simulink model "Pi_LUPA"  (R2024b)
settings: Solver=VariableStepAuto  StartTime=0.0  StopTime=t_stop  RelTol=1e-3
values from neighbouring files (symbols this model uses):
  C = 1.97e3/2    (= 985)    [general_pi_init.m]
  L = 5.21e-5    (= 5.21e-05)    [general_pi_init.m]
  SIL = sqrt(L/C)    [general_pi_init.m]
  T = table(freqs.', peak_ts.', peak_abk.', peak_conv.',      'VariableNames', {'Frequency_Hz','Peak_WAMIT_N','Peak_ABK_N','Peak_Conv_N'})    [F_ex_appx.m]    (also in general_pi_init.m = 10)
undefined symbols (not defined in the file or in its folder): A, ckt, dspblkCoreblockFVToolHelper, gcbh, IRF_dt, wd
libraries: fl_lib x229, nesl_utility x133, simulink x4, ee_lib x1
(part 1 of 4)
settings Model: Creator=inyongkim  LastModifiedBy=inyongkim

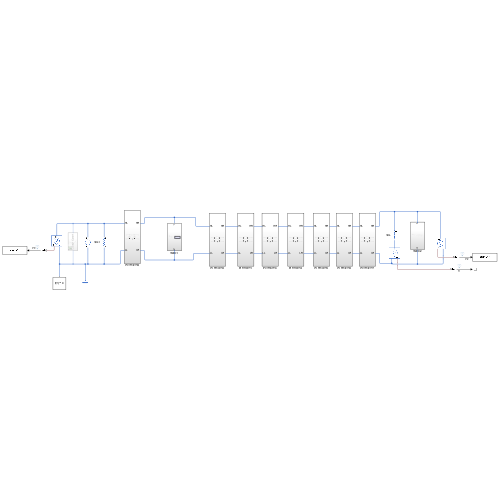
[thumbnail: Simulink's stored preview of the top-level diagram]
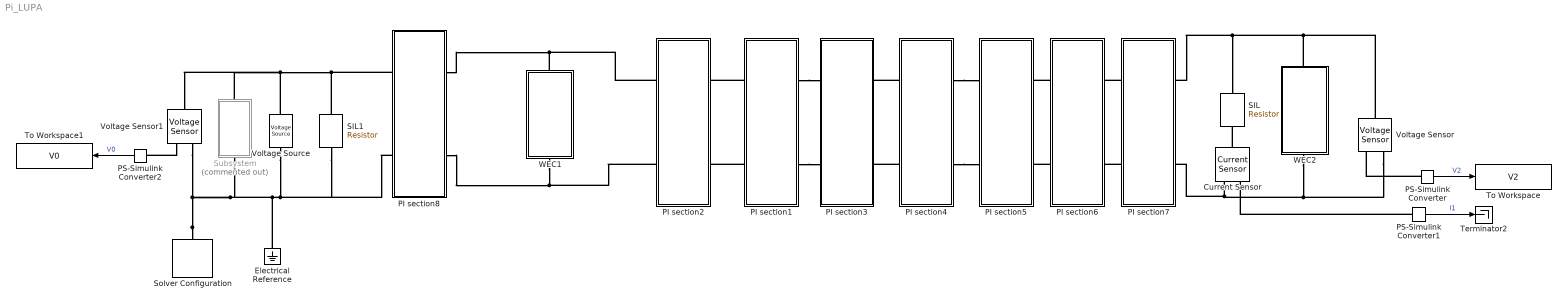
== system Pi_LUPA ==
  Current Sensor : fl_lib/Electrical/Electrical Sensors/Current Sensor
  Electrical Reference : fl_lib/Electrical/Electrical Elements/Electrical Reference
  PI section1 : Subsystem
  PI section2 : Subsystem
  PI section3 : Subsystem
  PI section4 : Subsystem
  PI section5 : Subsystem
  PI section6 : Subsystem
  PI section7 : Subsystem
  PI section8 : Subsystem
  PS-Simulink Converter : nesl_utility/PS-Simulink Converter  PhysicalDomain=network_engine_domain  SubClassName=ps_output  LeftPortType=input  RightPortType=output  PseudoPeriodic=off  Frequencies=[]  VectorFormat=inherit  Unit=inherit  AffineConversion=off
  PS-Simulink Converter1 : nesl_utility/PS-Simulink Converter  PhysicalDomain=network_engine_domain  SubClassName=ps_output  LeftPortType=input  RightPortType=output  PseudoPeriodic=off  Frequencies=[]  VectorFormat=inherit  Unit=inherit  AffineConversion=off
  PS-Simulink Converter2 : nesl_utility/PS-Simulink Converter  PhysicalDomain=network_engine_domain  SubClassName=ps_output  LeftPortType=input  RightPortType=output  PseudoPeriodic=off  Frequencies=[]  VectorFormat=inherit  Unit=inherit  AffineConversion=off
  SIL : fl_lib/Electrical/Electrical Elements/Resistor  R=SIL Ohm  i_specify=off  i_priority=None  i=0 A  i_nominal_specify=off  i_nominal_value=1  i_nominal_unit=A  v_specify=off  v_priority=None  v=0 V  v_nominal_specify=off  v_nominal_value=1  v_nominal_unit=V
  SIL1 : fl_lib/Electrical/Electrical Elements/Resistor  R=SIL*1e6 Ohm  i_specify=off  i_priority=None  i=0 A  i_nominal_specify=off  i_nominal_value=1  i_nominal_unit=A  v_specify=off  v_priority=None  v=0 V  v_nominal_specify=off  v_nominal_value=1  v_nominal_unit=V
  Solver Configuration : nesl_utility/Solver Configuration  PhysicalDomain=network_engine_domain  SubClassName=solver  LeftPortType=input  RightPortType=generic  Tones=[]  Harmonics=[]  SimulateNoise=off  Profile=off  UseLocalSampling=off  EnableSwitchedLinearOptims=on  FrequencyDomain=off  UseCCode=off  RelTol=0.001  AbsTol=0.001  MinStep=1e-09  ToWorkspace=off  RevertToSquareIcSolve=off  NumHomotopyIterations=100  PhasorMode=off  PhasorModeNumHarmonics=1  ConsistencySolver=NEWTON_XTOL_AFTER_FTOL  IndexReductionMethod=None  DoDC=off  ResidualTolerance=1e-09  ConsistencyTolSource=GLOBAL  ConsistencyAbsTol=0.001  ConsistencyRelTol=0.001  ConsistencyTolFactor=0.001  UseLocalSolver=off  LocalSolverChoice=NE_BACKWARD_EULER_ADVANCER  ResolveIndetEquations=on  FunctionEvalNumThread=1  LocalSolverSampleTime=0.001  DoFixedCost=off  MaxNonlinIter=3  MaxModeIter=2  ComputeImpulses=off  ImpulseIterations=2  LinearAlgebra=auto  LinearAlgebraNumThread=0  EquationFormulation=NE_TIME_EF  DelaysMemoryBudget=1024  AutomaticFiltering=on  FilteringTimeConstant=0.001  PartitionStorageMethod=AS_NEEDED  PartitionMemoryBudget=1024  PartitionMethod=ROBUST  MultibodyUseLocalSolver=off  MultibodyLocalSolverChoice=ODE1  MultibodyLocalSolverSampleTime=0.001
  Subsystem : Subsystem  Commented=on
  Terminator2 : Terminator
  To Workspace : ToWorkspace  VariableName=V2  SaveFormat=Timeseries  SampleTime=-1
  To Workspace1 : ToWorkspace  VariableName=V0  SaveFormat=Timeseries  SampleTime=-1
  Voltage Sensor : fl_lib/Electrical/Electrical Sensors/Voltage Sensor
  Voltage Sensor1 : fl_lib/Electrical/Electrical Sensors/Voltage Sensor
  Voltage Source : ee_lib/Sources/Voltage Source  dc_voltage=0 V  ac_voltage=A*2*pi/T V  ac_shift=0 rad  ac_frequency=1/T Hz  noise_mode=ee.enum.sources.noise.Disabled  PSD=0 V^2/Hz  sample_time=1e-3 s  repeatability=ee.enum.sources.repeatability.NotRepeatable  user_seed=0  auto_seed=3010019299  i_specify=off  i_priority=None  i=0 A  i_nominal_specify=off  i_nominal_value=1  i_nominal_unit=A  v_specify=off  v_priority=None  v=0 V  v_nominal_specify=off  v_nominal_value=1  v_nominal_unit=V
  WEC1 : Subsystem
      settings: PortSchema="{\"entries\":[{\"content\":{\"sides\":[{\"content\":{},\"type\":\"ConnectorPlacement.EquallySpacedRectSide\",\"uuid\":\"610af32e-2de7-4c50-99be-cfe133541e3f\"},{\"content\":{\"side\":\"RIGHT\"},\"type\":\"ConnectorPlacement.EquallySpacedRectSide\",\"uuid\":\"0415963f-e440-414e-b6ca-8ae2fc36710b\"},{\"content\":{\"connectorIds\":[\"LConn1\"],\"side\":\"TOP\"},\"type\":\"ConnectorPlacement.EquallySpacedRectSide\",\"uuid\":\"323fcf80-8c19-453d-8de3-ca4665704952\"},{\"content\":{\"connectorIds\":[\"RConn1\"],\"side\":\"BOTTOM\"},\"type\":\"ConnectorPlacement.EquallySpacedRectSide\",\"uuid\":\"a977eb3e-c443-4e6c-8731-998188d6bcfb\"}]},\"type\":\"ConnectorPlacement.EquallySpacedConnector\",\"uuid\":\"11f40d62-75d3-4550-8fc4-6982ab3d84ea\"}],\"packageUris\":[\"http://schema.mathworks.com/mf0/Connector/R2020b\"],\"version\":\"1.0\"}"
  WEC2 : Subsystem
      settings: PortSchema="{\"entries\":[{\"content\":{\"sides\":[{\"content\":{},\"type\":\"ConnectorPlacement.EquallySpacedRectSide\",\"uuid\":\"610af32e-2de7-4c50-99be-cfe133541e3f\"},{\"content\":{\"side\":\"RIGHT\"},\"type\":\"ConnectorPlacement.EquallySpacedRectSide\",\"uuid\":\"0415963f-e440-414e-b6ca-8ae2fc36710b\"},{\"content\":{\"connectorIds\":[\"LConn1\"],\"side\":\"TOP\"},\"type\":\"ConnectorPlacement.EquallySpacedRectSide\",\"uuid\":\"323fcf80-8c19-453d-8de3-ca4665704952\"},{\"content\":{\"connectorIds\":[\"RConn1\"],\"side\":\"BOTTOM\"},\"type\":\"ConnectorPlacement.EquallySpacedRectSide\",\"uuid\":\"a977eb3e-c443-4e6c-8731-998188d6bcfb\"}]},\"type\":\"ConnectorPlacement.EquallySpacedConnector\",\"uuid\":\"11f40d62-75d3-4550-8fc4-6982ab3d84ea\"}],\"packageUris\":[\"http://schema.mathworks.com/mf0/Connector/R2020b\"],\"version\":\"1.0\"}"
  wires:
  PS-Simulink Converter/1 -> To Workspace/1  "V2"
  PS-Simulink Converter1/1 -> Terminator2/1  "I1"
  PS-Simulink Converter2/1 -> To Workspace1/1  "V0"
  connections:
  Solver Configuration/RConn1 -- Subsystem/RConn1 -- Voltage Source/RConn1 -- SIL1/RConn1 -- PI section8/LConn2 -- Electrical Reference/LConn1 -- Voltage Sensor1/RConn2
  Voltage Source/LConn1 -- Subsystem/LConn1 -- Voltage Sensor1/LConn1 -- SIL1/LConn1 -- PI section8/LConn1
  Voltage Sensor/LConn1 -- WEC2/LConn1 -- SIL/LConn1 -- PI section7/RConn1
  PS-Simulink Converter/LConn1 -- Voltage Sensor/RConn1
  Current Sensor/LConn1 -- SIL/RConn1
  PS-Simulink Converter1/LConn1 -- Current Sensor/RConn1
  Voltage Sensor1/RConn1 -- PS-Simulink Converter2/LConn1
  WEC1/LConn1 -- PI section2/LConn1 -- PI section8/RConn1
  WEC1/RConn1 -- PI section2/LConn2 -- PI section8/RConn2
  Voltage Sensor/RConn2 -- WEC2/RConn1 -- PI section7/RConn2 -- Current Sensor/RConn2
  PI section1/RConn1 -- PI section3/LConn1
  PI section1/RConn2 -- PI section3/LConn2
  PI section4/LConn1 -- PI section3/RConn1
  PI section4/LConn2 -- PI section3/RConn2
  PI section4/RConn2 -- PI section5/LConn2
  PI section4/RConn1 -- PI section5/LConn1
  PI section6/LConn1 -- PI section5/RConn1
  PI section6/LConn2 -- PI section5/RConn2
  PI section1/LConn1 -- PI section2/RConn1
  PI section1/LConn2 -- PI section2/RConn2
  PI section7/LConn1 -- PI section6/RConn1
  PI section7/LConn2 -- PI section6/RConn2

== system Pi_LUPA/PI section1 ==
  Electrical Reference : fl_lib/Electrical/Electrical Elements/Electrical Reference
  General C : Subsystem
      settings: PortSchema="{\"entries\":[{\"content\":{\"sides\":[{\"content\":{},\"type\":\"ConnectorPlacement.EquallySpacedRectSide\",\"uuid\":\"54c7c027-76dd-4589-a14d-62021aaba10d\"},{\"content\":{\"side\":\"RIGHT\"},\"type\":\"ConnectorPlacement.EquallySpacedRectSide\",\"uuid\":\"5fae45fc-fbd0-44d0-9d3d-94b3e56c48e3\"},{\"content\":{\"connectorIds\":[\"LConn1\"],\"side\":\"TOP\"},\"type\":\"ConnectorPlacement.EquallySpacedRectSide\",\"uuid\":\"b6847d7e-9825-46ad-84aa-5df9156d119d\"},{\"content\":{\"connectorIds\":[\"RConn1\"],\"side\":\"BOTTOM\"},\"type\":\"ConnectorPlacement.EquallySpacedRectSide\",\"uuid\":\"1394d42d-8985-4309-a3e0-31ed6b8c9496\"}]},\"type\":\"ConnectorPlacement.EquallySpacedConnector\",\"uuid\":\"6a4af355-2598-47af-9220-e6e09375ad72\"}],\"packageUris\":[\"http://schema.mathworks.com/mf0/Connector/R2020b\"],\"version\":\"1.0\"}"
  General C1 : Subsystem
      settings: PortSchema="{\"entries\":[{\"content\":{\"sides\":[{\"content\":{},\"type\":\"ConnectorPlacement.EquallySpacedRectSide\",\"uuid\":\"54c7c027-76dd-4589-a14d-62021aaba10d\"},{\"content\":{\"side\":\"RIGHT\"},\"type\":\"ConnectorPlacement.EquallySpacedRectSide\",\"uuid\":\"5fae45fc-fbd0-44d0-9d3d-94b3e56c48e3\"},{\"content\":{\"connectorIds\":[\"LConn1\"],\"side\":\"TOP\"},\"type\":\"ConnectorPlacement.EquallySpacedRectSide\",\"uuid\":\"b6847d7e-9825-46ad-84aa-5df9156d119d\"},{\"content\":{\"connectorIds\":[\"RConn1\"],\"side\":\"BOTTOM\"},\"type\":\"ConnectorPlacement.EquallySpacedRectSide\",\"uuid\":\"1394d42d-8985-4309-a3e0-31ed6b8c9496\"}]},\"type\":\"ConnectorPlacement.EquallySpacedConnector\",\"uuid\":\"6a4af355-2598-47af-9220-e6e09375ad72\"}],\"packageUris\":[\"http://schema.mathworks.com/mf0/Connector/R2020b\"],\"version\":\"1.0\"}"
  General L : Subsystem
      settings: PortSchema="{\"entries\":[{\"content\":{\"sides\":[{\"content\":{},\"type\":\"ConnectorPlacement.EquallySpacedRectSide\",\"uuid\":\"54c7c027-76dd-4589-a14d-62021aaba10d\"},{\"content\":{\"side\":\"RIGHT\"},\"type\":\"ConnectorPlacement.EquallySpacedRectSide\",\"uuid\":\"5fae45fc-fbd0-44d0-9d3d-94b3e56c48e3\"},{\"content\":{\"connectorIds\":[\"LConn1\"],\"side\":\"TOP\"},\"type\":\"ConnectorPlacement.EquallySpacedRectSide\",\"uuid\":\"b6847d7e-9825-46ad-84aa-5df9156d119d\"},{\"content\":{\"connectorIds\":[\"RConn1\"],\"side\":\"BOTTOM\"},\"type\":\"ConnectorPlacement.EquallySpacedRectSide\",\"uuid\":\"7b301271-0a77-4acb-8843-591cb23b0585\"}]},\"type\":\"ConnectorPlacement.EquallySpacedConnector\",\"uuid\":\"6a4af355-2598-47af-9220-e6e09375ad72\"}],\"packageUris\":[\"http://schema.mathworks.com/mf0/Connector/R2020b\"],\"version\":\"1.0\"}"
  HL : PMIOPort  Side=Left
  HR : PMIOPort  Port=2  Side=Right
  LL : PMIOPort  Port=3  Side=Left
  LR : PMIOPort  Port=4  Side=Right
  connections:
  HL/RConn1 -- General L/LConn1 -- General C/LConn1
  General C/RConn1 -- LL/RConn1 -- Electrical Reference/LConn1 -- General C1/RConn1 -- LR/RConn1
  HR/RConn1 -- General C1/LConn1 -- General L/RConn1

== system Pi_LUPA/PI section2 ==
  Electrical Reference : fl_lib/Electrical/Electrical Elements/Electrical Reference
  General C : Subsystem
      settings: PortSchema="{\"entries\":[{\"content\":{\"sides\":[{\"content\":{},\"type\":\"ConnectorPlacement.EquallySpacedRectSide\",\"uuid\":\"54c7c027-76dd-4589-a14d-62021aaba10d\"},{\"content\":{\"side\":\"RIGHT\"},\"type\":\"ConnectorPlacement.EquallySpacedRectSide\",\"uuid\":\"5fae45fc-fbd0-44d0-9d3d-94b3e56c48e3\"},{\"content\":{\"connectorIds\":[\"LConn1\"],\"side\":\"TOP\"},\"type\":\"ConnectorPlacement.EquallySpacedRectSide\",\"uuid\":\"b6847d7e-9825-46ad-84aa-5df9156d119d\"},{\"content\":{\"connectorIds\":[\"RConn1\"],\"side\":\"BOTTOM\"},\"type\":\"ConnectorPlacement.EquallySpacedRectSide\",\"uuid\":\"1394d42d-8985-4309-a3e0-31ed6b8c9496\"}]},\"type\":\"ConnectorPlacement.EquallySpacedConnector\",\"uuid\":\"6a4af355-2598-47af-9220-e6e09375ad72\"}],\"packageUris\":[\"http://schema.mathworks.com/mf0/Connector/R2020b\"],\"version\":\"1.0\"}"
  General C1 : Subsystem
      settings: PortSchema="{\"entries\":[{\"content\":{\"sides\":[{\"content\":{},\"type\":\"ConnectorPlacement.EquallySpacedRectSide\",\"uuid\":\"54c7c027-76dd-4589-a14d-62021aaba10d\"},{\"content\":{\"side\":\"RIGHT\"},\"type\":\"ConnectorPlacement.EquallySpacedRectSide\",\"uuid\":\"5fae45fc-fbd0-44d0-9d3d-94b3e56c48e3\"},{\"content\":{\"connectorIds\":[\"LConn1\"],\"side\":\"TOP\"},\"type\":\"ConnectorPlacement.EquallySpacedRectSide\",\"uuid\":\"b6847d7e-9825-46ad-84aa-5df9156d119d\"},{\"content\":{\"connectorIds\":[\"RConn1\"],\"side\":\"BOTTOM\"},\"type\":\"ConnectorPlacement.EquallySpacedRectSide\",\"uuid\":\"1394d42d-8985-4309-a3e0-31ed6b8c9496\"}]},\"type\":\"ConnectorPlacement.EquallySpacedConnector\",\"uuid\":\"6a4af355-2598-47af-9220-e6e09375ad72\"}],\"packageUris\":[\"http://schema.mathworks.com/mf0/Connector/R2020b\"],\"version\":\"1.0\"}"
  General L : Subsystem
      settings: PortSchema="{\"entries\":[{\"content\":{\"sides\":[{\"content\":{},\"type\":\"ConnectorPlacement.EquallySpacedRectSide\",\"uuid\":\"54c7c027-76dd-4589-a14d-62021aaba10d\"},{\"content\":{\"side\":\"RIGHT\"},\"type\":\"ConnectorPlacement.EquallySpacedRectSide\",\"uuid\":\"5fae45fc-fbd0-44d0-9d3d-94b3e56c48e3\"},{\"content\":{\"connectorIds\":[\"LConn1\"],\"side\":\"TOP\"},\"type\":\"ConnectorPlacement.EquallySpacedRectSide\",\"uuid\":\"b6847d7e-9825-46ad-84aa-5df9156d119d\"},{\"content\":{\"connectorIds\":[\"RConn1\"],\"side\":\"BOTTOM\"},\"type\":\"ConnectorPlacement.EquallySpacedRectSide\",\"uuid\":\"7b301271-0a77-4acb-8843-591cb23b0585\"}]},\"type\":\"ConnectorPlacement.EquallySpacedConnector\",\"uuid\":\"6a4af355-2598-47af-9220-e6e09375ad72\"}],\"packageUris\":[\"http://schema.mathworks.com/mf0/Connector/R2020b\"],\"version\":\"1.0\"}"
  HL : PMIOPort  Side=Left
  HR : PMIOPort  Port=2  Side=Right
  LL : PMIOPort  Port=3  Side=Left
  LR : PMIOPort  Port=4  Side=Right
  connections:
  General L/RConn1 -- General C1/LConn1 -- HR/RConn1
  LR/RConn1 -- Electrical Reference/LConn1 -- LL/RConn1 -- General C/RConn1 -- General C1/RConn1
  General C/LConn1 -- General L/LConn1 -- HL/RConn1

== system Pi_LUPA/PI section3 ==
  Electrical Reference : fl_lib/Electrical/Electrical Elements/Electrical Reference
  General C : Subsystem
      settings: PortSchema="{\"entries\":[{\"content\":{\"sides\":[{\"content\":{},\"type\":\"ConnectorPlacement.EquallySpacedRectSide\",\"uuid\":\"54c7c027-76dd-4589-a14d-62021aaba10d\"},{\"content\":{\"side\":\"RIGHT\"},\"type\":\"ConnectorPlacement.EquallySpacedRectSide\",\"uuid\":\"5fae45fc-fbd0-44d0-9d3d-94b3e56c48e3\"},{\"content\":{\"connectorIds\":[\"LConn1\"],\"side\":\"TOP\"},\"type\":\"ConnectorPlacement.EquallySpacedRectSide\",\"uuid\":\"b6847d7e-9825-46ad-84aa-5df9156d119d\"},{\"content\":{\"connectorIds\":[\"RConn1\"],\"side\":\"BOTTOM\"},\"type\":\"ConnectorPlacement.EquallySpacedRectSide\",\"uuid\":\"1394d42d-8985-4309-a3e0-31ed6b8c9496\"}]},\"type\":\"ConnectorPlacement.EquallySpacedConnector\",\"uuid\":\"6a4af355-2598-47af-9220-e6e09375ad72\"}],\"packageUris\":[\"http://schema.mathworks.com/mf0/Connector/R2020b\"],\"version\":\"1.0\"}"
  General C1 : Subsystem
      settings: PortSchema="{\"entries\":[{\"content\":{\"sides\":[{\"content\":{},\"type\":\"ConnectorPlacement.EquallySpacedRectSide\",\"uuid\":\"54c7c027-76dd-4589-a14d-62021aaba10d\"},{\"content\":{\"side\":\"RIGHT\"},\"type\":\"ConnectorPlacement.EquallySpacedRectSide\",\"uuid\":\"5fae45fc-fbd0-44d0-9d3d-94b3e56c48e3\"},{\"content\":{\"connectorIds\":[\"LConn1\"],\"side\":\"TOP\"},\"type\":\"ConnectorPlacement.EquallySpacedRectSide\",\"uuid\":\"b6847d7e-9825-46ad-84aa-5df9156d119d\"},{\"content\":{\"connectorIds\":[\"RConn1\"],\"side\":\"BOTTOM\"},\"type\":\"ConnectorPlacement.EquallySpacedRectSide\",\"uuid\":\"1394d42d-8985-4309-a3e0-31ed6b8c9496\"}]},\"type\":\"ConnectorPlacement.EquallySpacedConnector\",\"uuid\":\"6a4af355-2598-47af-9220-e6e09375ad72\"}],\"packageUris\":[\"http://schema.mathworks.com/mf0/Connector/R2020b\"],\"version\":\"1.0\"}"
  General L : Subsystem
      settings: PortSchema="{\"entries\":[{\"content\":{\"sides\":[{\"content\":{},\"type\":\"ConnectorPlacement.EquallySpacedRectSide\",\"uuid\":\"54c7c027-76dd-4589-a14d-62021aaba10d\"},{\"content\":{\"side\":\"RIGHT\"},\"type\":\"ConnectorPlacement.EquallySpacedRectSide\",\"uuid\":\"5fae45fc-fbd0-44d0-9d3d-94b3e56c48e3\"},{\"content\":{\"connectorIds\":[\"LConn1\"],\"side\":\"TOP\"},\"type\":\"ConnectorPlacement.EquallySpacedRectSide\",\"uuid\":\"b6847d7e-9825-46ad-84aa-5df9156d119d\"},{\"content\":{\"connectorIds\":[\"RConn1\"],\"side\":\"BOTTOM\"},\"type\":\"ConnectorPlacement.EquallySpacedRectSide\",\"uuid\":\"7b301271-0a77-4acb-8843-591cb23b0585\"}]},\"type\":\"ConnectorPlacement.EquallySpacedConnector\",\"uuid\":\"6a4af355-2598-47af-9220-e6e09375ad72\"}],\"packageUris\":[\"http://schema.mathworks.com/mf0/Connector/R2020b\"],\"version\":\"1.0\"}"
  HL : PMIOPort  Side=Left
  HR : PMIOPort  Port=2  Side=Right
  LL : PMIOPort  Port=3  Side=Left
  LR : PMIOPort  Port=4  Side=Right
  connections:
  General L/RConn1 -- General C1/LConn1 -- HR/RConn1
  LR/RConn1 -- Electrical Reference/LConn1 -- LL/RConn1 -- General C/RConn1 -- General C1/RConn1
  General C/LConn1 -- General L/LConn1 -- HL/RConn1

== system Pi_LUPA/PI section4 ==
  Electrical Reference : fl_lib/Electrical/Electrical Elements/Electrical Reference
  General C : Subsystem
      settings: PortSchema="{\"entries\":[{\"content\":{\"sides\":[{\"content\":{},\"type\":\"ConnectorPlacement.EquallySpacedRectSide\",\"uuid\":\"54c7c027-76dd-4589-a14d-62021aaba10d\"},{\"content\":{\"side\":\"RIGHT\"},\"type\":\"ConnectorPlacement.EquallySpacedRectSide\",\"uuid\":\"5fae45fc-fbd0-44d0-9d3d-94b3e56c48e3\"},{\"content\":{\"connectorIds\":[\"LConn1\"],\"side\":\"TOP\"},\"type\":\"ConnectorPlacement.EquallySpacedRectSide\",\"uuid\":\"b6847d7e-9825-46ad-84aa-5df9156d119d\"},{\"content\":{\"connectorIds\":[\"RConn1\"],\"side\":\"BOTTOM\"},\"type\":\"ConnectorPlacement.EquallySpacedRectSide\",\"uuid\":\"1394d42d-8985-4309-a3e0-31ed6b8c9496\"}]},\"type\":\"ConnectorPlacement.EquallySpacedConnector\",\"uuid\":\"6a4af355-2598-47af-9220-e6e09375ad72\"}],\"packageUris\":[\"http://schema.mathworks.com/mf0/Connector/R2020b\"],\"version\":\"1.0\"}"
  General C1 : Subsystem
      settings: PortSchema="{\"entries\":[{\"content\":{\"sides\":[{\"content\":{},\"type\":\"ConnectorPlacement.EquallySpacedRectSide\",\"uuid\":\"54c7c027-76dd-4589-a14d-62021aaba10d\"},{\"content\":{\"side\":\"RIGHT\"},\"type\":\"ConnectorPlacement.EquallySpacedRectSide\",\"uuid\":\"5fae45fc-fbd0-44d0-9d3d-94b3e56c48e3\"},{\"content\":{\"connectorIds\":[\"LConn1\"],\"side\":\"TOP\"},\"type\":\"ConnectorPlacement.EquallySpacedRectSide\",\"uuid\":\"b6847d7e-9825-46ad-84aa-5df9156d119d\"},{\"content\":{\"connectorIds\":[\"RConn1\"],\"side\":\"BOTTOM\"},\"type\":\"ConnectorPlacement.EquallySpacedRectSide\",\"uuid\":\"1394d42d-8985-4309-a3e0-31ed6b8c9496\"}]},\"type\":\"ConnectorPlacement.EquallySpacedConnector\",\"uuid\":\"6a4af355-2598-47af-9220-e6e09375ad72\"}],\"packageUris\":[\"http://schema.mathworks.com/mf0/Connector/R2020b\"],\"version\":\"1.0\"}"
  General L : Subsystem
      settings: PortSchema="{\"entries\":[{\"content\":{\"sides\":[{\"content\":{},\"type\":\"ConnectorPlacement.EquallySpacedRectSide\",\"uuid\":\"54c7c027-76dd-4589-a14d-62021aaba10d\"},{\"content\":{\"side\":\"RIGHT\"},\"type\":\"ConnectorPlacement.EquallySpacedRectSide\",\"uuid\":\"5fae45fc-fbd0-44d0-9d3d-94b3e56c48e3\"},{\"content\":{\"connectorIds\":[\"LConn1\"],\"side\":\"TOP\"},\"type\":\"ConnectorPlacement.EquallySpacedRectSide\",\"uuid\":\"b6847d7e-9825-46ad-84aa-5df9156d119d\"},{\"content\":{\"connectorIds\":[\"RConn1\"],\"side\":\"BOTTOM\"},\"type\":\"ConnectorPlacement.EquallySpacedRectSide\",\"uuid\":\"7b301271-0a77-4acb-8843-591cb23b0585\"}]},\"type\":\"ConnectorPlacement.EquallySpacedConnector\",\"uuid\":\"6a4af355-2598-47af-9220-e6e09375ad72\"}],\"packageUris\":[\"http://schema.mathworks.com/mf0/Connector/R2020b\"],\"version\":\"1.0\"}"
  HL : PMIOPort  Side=Left
  HR : PMIOPort  Port=2  Side=Right
  LL : PMIOPort  Port=3  Side=Left
  LR : PMIOPort  Port=4  Side=Right
  connections:
  General L/RConn1 -- General C1/LConn1 -- HR/RConn1
  LR/RConn1 -- Electrical Reference/LConn1 -- LL/RConn1 -- General C/RConn1 -- General C1/RConn1
  General C/LConn1 -- General L/LConn1 -- HL/RConn1

== system Pi_LUPA/PI section5 ==
  Electrical Reference : fl_lib/Electrical/Electrical Elements/Electrical Reference
  General C : Subsystem
      settings: PortSchema="{\"entries\":[{\"content\":{\"sides\":[{\"content\":{},\"type\":\"ConnectorPlacement.EquallySpacedRectSide\",\"uuid\":\"54c7c027-76dd-4589-a14d-62021aaba10d\"},{\"content\":{\"side\":\"RIGHT\"},\"type\":\"ConnectorPlacement.EquallySpacedRectSide\",\"uuid\":\"5fae45fc-fbd0-44d0-9d3d-94b3e56c48e3\"},{\"content\":{\"connectorIds\":[\"LConn1\"],\"side\":\"TOP\"},\"type\":\"ConnectorPlacement.EquallySpacedRectSide\",\"uuid\":\"b6847d7e-9825-46ad-84aa-5df9156d119d\"},{\"content\":{\"connectorIds\":[\"RConn1\"],\"side\":\"BOTTOM\"},\"type\":\"ConnectorPlacement.EquallySpacedRectSide\",\"uuid\":\"1394d42d-8985-4309-a3e0-31ed6b8c9496\"}]},\"type\":\"ConnectorPlacement.EquallySpacedConnector\",\"uuid\":\"6a4af355-2598-47af-9220-e6e09375ad72\"}],\"packageUris\":[\"http://schema.mathworks.com/mf0/Connector/R2020b\"],\"version\":\"1.0\"}"
  General C1 : Subsystem
      settings: PortSchema="{\"entries\":[{\"content\":{\"sides\":[{\"content\":{},\"type\":\"ConnectorPlacement.EquallySpacedRectSide\",\"uuid\":\"54c7c027-76dd-4589-a14d-62021aaba10d\"},{\"content\":{\"side\":\"RIGHT\"},\"type\":\"ConnectorPlacement.EquallySpacedRectSide\",\"uuid\":\"5fae45fc-fbd0-44d0-9d3d-94b3e56c48e3\"},{\"content\":{\"connectorIds\":[\"LConn1\"],\"side\":\"TOP\"},\"type\":\"ConnectorPlacement.EquallySpacedRectSide\",\"uuid\":\"b6847d7e-9825-46ad-84aa-5df9156d119d\"},{\"content\":{\"connectorIds\":[\"RConn1\"],\"side\":\"BOTTOM\"},\"type\":\"ConnectorPlacement.EquallySpacedRectSide\",\"uuid\":\"1394d42d-8985-4309-a3e0-31ed6b8c9496\"}]},\"type\":\"ConnectorPlacement.EquallySpacedConnector\",\"uuid\":\"6a4af355-2598-47af-9220-e6e09375ad72\"}],\"packageUris\":[\"http://schema.mathworks.com/mf0/Connector/R2020b\"],\"version\":\"1.0\"}"
  General L : Subsystem
      settings: PortSchema="{\"entries\":[{\"content\":{\"sides\":[{\"content\":{},\"type\":\"ConnectorPlacement.EquallySpacedRectSide\",\"uuid\":\"54c7c027-76dd-4589-a14d-62021aaba10d\"},{\"content\":{\"side\":\"RIGHT\"},\"type\":\"ConnectorPlacement.EquallySpacedRectSide\",\"uuid\":\"5fae45fc-fbd0-44d0-9d3d-94b3e56c48e3\"},{\"content\":{\"connectorIds\":[\"LConn1\"],\"side\":\"TOP\"},\"type\":\"ConnectorPlacement.EquallySpacedRectSide\",\"uuid\":\"b6847d7e-9825-46ad-84aa-5df9156d119d\"},{\"content\":{\"connectorIds\":[\"RConn1\"],\"side\":\"BOTTOM\"},\"type\":\"ConnectorPlacement.EquallySpacedRectSide\",\"uuid\":\"7b301271-0a77-4acb-8843-591cb23b0585\"}]},\"type\":\"ConnectorPlacement.EquallySpacedConnector\",\"uuid\":\"6a4af355-2598-47af-9220-e6e09375ad72\"}],\"packageUris\":[\"http://schema.mathworks.com/mf0/Connector/R2020b\"],\"version\":\"1.0\"}"
  HL : PMIOPort  Side=Left
  HR : PMIOPort  Port=2  Side=Right
  LL : PMIOPort  Port=3  Side=Left
  LR : PMIOPort  Port=4  Side=Right
  connections:
  HL/RConn1 -- General L/LConn1 -- General C/LConn1
  General C/RConn1 -- LL/RConn1 -- Electrical Reference/LConn1 -- General C1/RConn1 -- LR/RConn1
  HR/RConn1 -- General C1/LConn1 -- General L/RConn1

== system Pi_LUPA/PI section6 ==
  Electrical Reference : fl_lib/Electrical/Electrical Elements/Electrical Reference
  General C : Subsystem
      settings: PortSchema="{\"entries\":[{\"content\":{\"sides\":[{\"content\":{},\"type\":\"ConnectorPlacement.EquallySpacedRectSide\",\"uuid\":\"54c7c027-76dd-4589-a14d-62021aaba10d\"},{\"content\":{\"side\":\"RIGHT\"},\"type\":\"ConnectorPlacement.EquallySpacedRectSide\",\"uuid\":\"5fae45fc-fbd0-44d0-9d3d-94b3e56c48e3\"},{\"content\":{\"connectorIds\":[\"LConn1\"],\"side\":\"TOP\"},\"type\":\"ConnectorPlacement.EquallySpacedRectSide\",\"uuid\":\"b6847d7e-9825-46ad-84aa-5df9156d119d\"},{\"content\":{\"connectorIds\":[\"RConn1\"],\"side\":\"BOTTOM\"},\"type\":\"ConnectorPlacement.EquallySpacedRectSide\",\"uuid\":\"1394d42d-8985-4309-a3e0-31ed6b8c9496\"}]},\"type\":\"ConnectorPlacement.EquallySpacedConnector\",\"uuid\":\"6a4af355-2598-47af-9220-e6e09375ad72\"}],\"packageUris\":[\"http://schema.mathworks.com/mf0/Connector/R2020b\"],\"version\":\"1.0\"}"
  General C1 : Subsystem
      settings: PortSchema="{\"entries\":[{\"content\":{\"sides\":[{\"content\":{},\"type\":\"ConnectorPlacement.EquallySpacedRectSide\",\"uuid\":\"54c7c027-76dd-4589-a14d-62021aaba10d\"},{\"content\":{\"side\":\"RIGHT\"},\"type\":\"ConnectorPlacement.EquallySpacedRectSide\",\"uuid\":\"5fae45fc-fbd0-44d0-9d3d-94b3e56c48e3\"},{\"content\":{\"connectorIds\":[\"LConn1\"],\"side\":\"TOP\"},\"type\":\"ConnectorPlacement.EquallySpacedRectSide\",\"uuid\":\"b6847d7e-9825-46ad-84aa-5df9156d119d\"},{\"content\":{\"connectorIds\":[\"RConn1\"],\"side\":\"BOTTOM\"},\"type\":\"ConnectorPlacement.EquallySpacedRectSide\",\"uuid\":\"1394d42d-8985-4309-a3e0-31ed6b8c9496\"}]},\"type\":\"ConnectorPlacement.EquallySpacedConnector\",\"uuid\":\"6a4af355-2598-47af-9220-e6e09375ad72\"}],\"packageUris\":[\"http://schema.mathworks.com/mf0/Connector/R2020b\"],\"version\":\"1.0\"}"
  General L : Subsystem
      settings: PortSchema="{\"entries\":[{\"content\":{\"sides\":[{\"content\":{},\"type\":\"ConnectorPlacement.EquallySpacedRectSide\",\"uuid\":\"54c7c027-76dd-4589-a14d-62021aaba10d\"},{\"content\":{\"side\":\"RIGHT\"},\"type\":\"ConnectorPlacement.EquallySpacedRectSide\",\"uuid\":\"5fae45fc-fbd0-44d0-9d3d-94b3e56c48e3\"},{\"content\":{\"connectorIds\":[\"LConn1\"],\"side\":\"TOP\"},\"type\":\"ConnectorPlacement.EquallySpacedRectSide\",\"uuid\":\"b6847d7e-9825-46ad-84aa-5df9156d119d\"},{\"content\":{\"connectorIds\":[\"RConn1\"],\"side\":\"BOTTOM\"},\"type\":\"ConnectorPlacement.EquallySpacedRectSide\",\"uuid\":\"7b301271-0a77-4acb-8843-591cb23b0585\"}]},\"type\":\"ConnectorPlacement.EquallySpacedConnector\",\"uuid\":\"6a4af355-2598-47af-9220-e6e09375ad72\"}],\"packageUris\":[\"http://schema.mathworks.com/mf0/Connector/R2020b\"],\"version\":\"1.0\"}"
  HL : PMIOPort  Side=Left
  HR : PMIOPort  Port=2  Side=Right
  LL : PMIOPort  Port=3  Side=Left
  LR : PMIOPort  Port=4  Side=Right
  connections:
  General L/RConn1 -- General C1/LConn1 -- HR/RConn1
  LR/RConn1 -- Electrical Reference/LConn1 -- LL/RConn1 -- General C/RConn1 -- General C1/RConn1
  General C/LConn1 -- General L/LConn1 -- HL/RConn1

== system Pi_LUPA/PI section7 ==
  Electrical Reference : fl_lib/Electrical/Electrical Elements/Electrical Reference
  General C : Subsystem
      settings: PortSchema="{\"entries\":[{\"content\":{\"sides\":[{\"content\":{},\"type\":\"ConnectorPlacement.EquallySpacedRectSide\",\"uuid\":\"54c7c027-76dd-4589-a14d-62021aaba10d\"},{\"content\":{\"side\":\"RIGHT\"},\"type\":\"ConnectorPlacement.EquallySpacedRectSide\",\"uuid\":\"5fae45fc-fbd0-44d0-9d3d-94b3e56c48e3\"},{\"content\":{\"connectorIds\":[\"LConn1\"],\"side\":\"TOP\"},\"type\":\"ConnectorPlacement.EquallySpacedRectSide\",\"uuid\":\"b6847d7e-9825-46ad-84aa-5df9156d119d\"},{\"content\":{\"connectorIds\":[\"RConn1\"],\"side\":\"BOTTOM\"},\"type\":\"ConnectorPlacement.EquallySpacedRectSide\",\"uuid\":\"1394d42d-8985-4309-a3e0-31ed6b8c9496\"}]},\"type\":\"ConnectorPlacement.EquallySpacedConnector\",\"uuid\":\"6a4af355-2598-47af-9220-e6e09375ad72\"}],\"packageUris\":[\"http://schema.mathworks.com/mf0/Connector/R2020b\"],\"version\":\"1.0\"}"
  General C1 : Subsystem
      settings: PortSchema="{\"entries\":[{\"content\":{\"sides\":[{\"content\":{},\"type\":\"ConnectorPlacement.EquallySpacedRectSide\",\"uuid\":\"54c7c027-76dd-4589-a14d-62021aaba10d\"},{\"content\":{\"side\":\"RIGHT\"},\"type\":\"ConnectorPlacement.EquallySpacedRectSide\",\"uuid\":\"5fae45fc-fbd0-44d0-9d3d-94b3e56c48e3\"},{\"content\":{\"connectorIds\":[\"LConn1\"],\"side\":\"TOP\"},\"type\":\"ConnectorPlacement.EquallySpacedRectSide\",\"uuid\":\"b6847d7e-9825-46ad-84aa-5df9156d119d\"},{\"content\":{\"connectorIds\":[\"RConn1\"],\"side\":\"BOTTOM\"},\"type\":\"ConnectorPlacement.EquallySpacedRectSide\",\"uuid\":\"1394d42d-8985-4309-a3e0-31ed6b8c9496\"}]},\"type\":\"ConnectorPlacement.EquallySpacedConnector\",\"uuid\":\"6a4af355-2598-47af-9220-e6e09375ad72\"}],\"packageUris\":[\"http://schema.mathworks.com/mf0/Connector/R2020b\"],\"version\":\"1.0\"}"
  General L : Subsystem
      settings: PortSchema="{\"entries\":[{\"content\":{\"sides\":[{\"content\":{},\"type\":\"ConnectorPlacement.EquallySpacedRectSide\",\"uuid\":\"54c7c027-76dd-4589-a14d-62021aaba10d\"},{\"content\":{\"side\":\"RIGHT\"},\"type\":\"ConnectorPlacement.EquallySpacedRectSide\",\"uuid\":\"5fae45fc-fbd0-44d0-9d3d-94b3e56c48e3\"},{\"content\":{\"connectorIds\":[\"LConn1\"],\"side\":\"TOP\"},\"type\":\"ConnectorPlacement.EquallySpacedRectSide\",\"uuid\":\"b6847d7e-9825-46ad-84aa-5df9156d119d\"},{\"content\":{\"connectorIds\":[\"RConn1\"],\"side\":\"BOTTOM\"},\"type\":\"ConnectorPlacement.EquallySpacedRectSide\",\"uuid\":\"7b301271-0a77-4acb-8843-591cb23b0585\"}]},\"type\":\"ConnectorPlacement.EquallySpacedConnector\",\"uuid\":\"6a4af355-2598-47af-9220-e6e09375ad72\"}],\"packageUris\":[\"http://schema.mathworks.com/mf0/Connector/R2020b\"],\"version\":\"1.0\"}"
  HL : PMIOPort  Side=Left
  HR : PMIOPort  Port=2  Side=Right
  LL : PMIOPort  Port=3  Side=Left
  LR : PMIOPort  Port=4  Side=Right
  connections:
  HL/RConn1 -- General L/LConn1 -- General C/LConn1
  General C/RConn1 -- LL/RConn1 -- Electrical Reference/LConn1 -- General C1/RConn1 -- LR/RConn1
  HR/RConn1 -- General C1/LConn1 -- General L/RConn1

== system Pi_LUPA/PI section8 ==
  Electrical Reference : fl_lib/Electrical/Electrical Elements/Electrical Reference
  General C : Subsystem
      settings: PortSchema="{\"entries\":[{\"content\":{\"sides\":[{\"content\":{},\"type\":\"ConnectorPlacement.EquallySpacedRectSide\",\"uuid\":\"54c7c027-76dd-4589-a14d-62021aaba10d\"},{\"content\":{\"side\":\"RIGHT\"},\"type\":\"ConnectorPlacement.EquallySpacedRectSide\",\"uuid\":\"5fae45fc-fbd0-44d0-9d3d-94b3e56c48e3\"},{\"content\":{\"connectorIds\":[\"LConn1\"],\"side\":\"TOP\"},\"type\":\"ConnectorPlacement.EquallySpacedRectSide\",\"uuid\":\"b6847d7e-9825-46ad-84aa-5df9156d119d\"},{\"content\":{\"connectorIds\":[\"RConn1\"],\"side\":\"BOTTOM\"},\"type\":\"ConnectorPlacement.EquallySpacedRectSide\",\"uuid\":\"1394d42d-8985-4309-a3e0-31ed6b8c9496\"}]},\"type\":\"ConnectorPlacement.EquallySpacedConnector\",\"uuid\":\"6a4af355-2598-47af-9220-e6e09375ad72\"}],\"packageUris\":[\"http://schema.mathworks.com/mf0/Connector/R2020b\"],\"version\":\"1.0\"}"
  General C1 : Subsystem
      settings: PortSchema="{\"entries\":[{\"content\":{\"sides\":[{\"content\":{},\"type\":\"ConnectorPlacement.EquallySpacedRectSide\",\"uuid\":\"54c7c027-76dd-4589-a14d-62021aaba10d\"},{\"content\":{\"side\":\"RIGHT\"},\"type\":\"ConnectorPlacement.EquallySpacedRectSide\",\"uuid\":\"5fae45fc-fbd0-44d0-9d3d-94b3e56c48e3\"},{\"content\":{\"connectorIds\":[\"LConn1\"],\"side\":\"TOP\"},\"type\":\"ConnectorPlacement.EquallySpacedRectSide\",\"uuid\":\"b6847d7e-9825-46ad-84aa-5df9156d119d\"},{\"content\":{\"connectorIds\":[\"RConn1\"],\"side\":\"BOTTOM\"},\"type\":\"ConnectorPlacement.EquallySpacedRectSide\",\"uuid\":\"1394d42d-8985-4309-a3e0-31ed6b8c9496\"}]},\"type\":\"ConnectorPlacement.EquallySpacedConnector\",\"uuid\":\"6a4af355-2598-47af-9220-e6e09375ad72\"}],\"packageUris\":[\"http://schema.mathworks.com/mf0/Connector/R2020b\"],\"version\":\"1.0\"}"
  General L : Subsystem
      settings: PortSchema="{\"entries\":[{\"content\":{\"sides\":[{\"content\":{},\"type\":\"ConnectorPlacement.EquallySpacedRectSide\",\"uuid\":\"54c7c027-76dd-4589-a14d-62021aaba10d\"},{\"content\":{\"side\":\"RIGHT\"},\"type\":\"ConnectorPlacement.EquallySpacedRectSide\",\"uuid\":\"5fae45fc-fbd0-44d0-9d3d-94b3e56c48e3\"},{\"content\":{\"connectorIds\":[\"LConn1\"],\"side\":\"TOP\"},\"type\":\"ConnectorPlacement.EquallySpacedRectSide\",\"uuid\":\"b6847d7e-9825-46ad-84aa-5df9156d119d\"},{\"content\":{\"connectorIds\":[\"RConn1\"],\"side\":\"BOTTOM\"},\"type\":\"ConnectorPlacement.EquallySpacedRectSide\",\"uuid\":\"7b301271-0a77-4acb-8843-591cb23b0585\"}]},\"type\":\"ConnectorPlacement.EquallySpacedConnector\",\"uuid\":\"6a4af355-2598-47af-9220-e6e09375ad72\"}],\"packageUris\":[\"http://schema.mathworks.com/mf0/Connector/R2020b\"],\"version\":\"1.0\"}"
  HL : PMIOPort  Side=Left
  HR : PMIOPort  Port=2  Side=Right
  LL : PMIOPort  Port=3  Side=Left
  LR : PMIOPort  Port=4  Side=Right
  connections:
  General L/RConn1 -- General C1/LConn1 -- HR/RConn1
  LR/RConn1 -- Electrical Reference/LConn1 -- LL/RConn1 -- General C/RConn1 -- General C1/RConn1
  General C/LConn1 -- General L/LConn1 -- HL/RConn1

== system Pi_LUPA/Subsystem ==
  Controlled Voltage Source : fl_lib/Electrical/Electrical Sources/Controlled Voltage Source
  Gain : Gain  Gain=1/T*pi*2
  Product : Product
  Ramp : simulink/Sources/Ramp  slope=1/4/T  start=0  InitialOutput=0
  Ramp1 : simulink/Sources/Ramp  slope=1  start=0  InitialOutput=0
  Saturation : Saturate  UpperLimit=0.1  LowerLimit=0
  Simulink-PS Converter : nesl_utility/Simulink-PS Converter  PhysicalDomain=network_engine_domain  SubClassName=ps_input  LeftPortType=input  RightPortType=output  PseudoPeriodic=off  Frequencies=[]  NoiseDistribution=none  NoiseParameters=[]  Unit=V  AffineConversion=off  FilteringAndDerivatives=provide  SimscapeFilterOrder=1  InputFilterTimeConstant=0.001  UdotUserProvided=0
  Trigonometric Function : Trigonometry
  Conn1 : PMIOPort  Side=Left
  Conn2 : PMIOPort  Port=2  Side=Right
  wires:
  Gain/1 -> Trigonometric Function/1
  Ramp/1 -> Saturation/1
  Ramp1/1 -> Gain/1
  Saturation/1 -> Product/1
  Trigonometric Function/1 -> Product/2
  Product/1 -> Simulink-PS Converter/1  "V0"
  connections:
  Controlled Voltage Source/LConn1 -- Conn1/RConn1
  Controlled Voltage Source/RConn2 -- Conn2/RConn1
  Simulink-PS Converter/RConn1 -- Controlled Voltage Source/RConn1

== system Pi_LUPA/WEC1 ==
  note: LUPA1
  Add : Sum  Inputs=+++
  B_rad : Gain  Gain=1/ckt.R_rad
  Capacitor1 : fl_lib/Electrical/Electrical Elements/Capacitor  c=ckt.C_M F  r=0 Ohm  g=0 1/Ohm  i_specify=off  i_priority=None  i=0 A  i_nominal_specify=off  i_nominal_value=1  i_nominal_unit=A  v_specify=off  v_priority=None  v=0 V  v_nominal_specify=off  v_nominal_value=1  v_nominal_unit=V  vc_specify=off  vc_priority=High  vc=0 V  vc_nominal_specify=off  vc_nominal_value=1  vc_nominal_unit=V
  Controlled Current Source : fl_lib/Electrical/Electrical Sources/Controlled Current Source
  Divide : Product  Commented=on  Inputs=*/
  Electrical Reference : fl_lib/Electrical/Electrical Elements/Electrical Reference
  Electrical Reference2 : fl_lib/Electrical/Electrical Elements/Electrical Reference
  Fex_FIR_IRF : Subsystem  Commented=on
  Gain : Gain  Gain=0.65
  Inductor1 : fl_lib/Electrical/Electrical Elements/Inductor  l=ckt.L_hs H  r=0 Ohm  g=0 1/Ohm  i_specify=off  i_priority=None  i=0 A  i_nominal_specify=off  i_nominal_value=1  i_nominal_unit=A  v_specify=off  v_priority=None  v=0 V  v_nominal_specify=off  v_nominal_value=1  v_nominal_unit=V  i_L_specify=off  i_L_priority=High  i_L=0 A  i_L_nominal_specify=off  i_L_nominal_value=1  i_L_nominal_unit=A
  Integrator : Integrator  InitialCondition=-A
  K_hs : Gain  Gain=1/ckt.L_hs
  M_add : Gain  Gain=ckt.C_add
  PS-Simulink Converter : nesl_utility/PS-Simulink Converter  PhysicalDomain=network_engine_domain  SubClassName=ps_output  LeftPortType=input  RightPortType=output  PseudoPeriodic=off  Frequencies=[]  VectorFormat=inherit  Unit=inherit  AffineConversion=off
  PS-Simulink Converter1 : nesl_utility/PS-Simulink Converter  PhysicalDomain=network_engine_domain  SubClassName=ps_output  LeftPortType=input  RightPortType=output  PseudoPeriodic=off  Frequencies=[]  VectorFormat=inherit  Unit=V  AffineConversion=off
  Product : Product
  Resistor : fl_lib/Electrical/Electrical Elements/Resistor  R=1.1*1e-3 Ohm  i_specify=off  i_priority=None  i=0 A  i_nominal_specify=off  i_nominal_value=1  i_nominal_unit=A  v_specify=off  v_priority=None  v=0 V  v_nominal_specify=off  v_nominal_value=1  v_nominal_unit=V
  Resistor1 : fl_lib/Electrical/Electrical Elements/Resistor  R=ckt.R_rad Ohm  i_specify=off  i_priority=None  i=0 A  i_nominal_specify=off  i_nominal_value=1  i_nominal_unit=A  v_specify=off  v_priority=None  v=0 V  v_nominal_specify=off  v_nominal_value=1  v_nominal_unit=V
  Resistor2 : fl_lib/Electrical/Electrical Elements/Resistor  R=ckt.R_fric Ohm  i_specify=off  i_priority=None  i=0 A  i_nominal_specify=off  i_nominal_value=1  i_nominal_unit=A  v_specify=off  v_priority=None  v=0 V  v_nominal_specify=off  v_nominal_value=1  v_nominal_unit=V
  Resistor3 : fl_lib/Electrical/Electrical Elements/Resistor  R=ckt.R_pto Ohm  i_specify=off  i_priority=None  i=0 A  i_nominal_specify=off  i_nominal_value=1  i_nominal_unit=A  v_specify=off  v_priority=None  v=0 V  v_nominal_specify=off  v_nominal_value=1  v_nominal_unit=V
  Simulink-PS Converter : nesl_utility/Simulink-PS Converter  PhysicalDomain=network_engine_domain  SubClassName=ps_input  LeftPortType=input  RightPortType=output  PseudoPeriodic=off  Frequencies=[]  NoiseDistribution=none  NoiseParameters=[]  Unit=A  AffineConversion=off  FilteringAndDerivatives=filter  SimscapeFilterOrder=1  InputFilterTimeConstant=0.001  UdotUserProvided=0
  Solver Configuration : nesl_utility/Solver Configuration  PhysicalDomain=network_engine_domain  SubClassName=solver  LeftPortType=input  RightPortType=generic  Tones=[]  Harmonics=[]  SimulateNoise=off  Profile=off  UseLocalSampling=off  EnableSwitchedLinearOptims=on  FrequencyDomain=off  UseCCode=off  RelTol=0.001  AbsTol=0.001  MinStep=1e-09  ToWorkspace=off  RevertToSquareIcSolve=off  NumHomotopyIterations=100  PhasorMode=off  PhasorModeNumHarmonics=1  ConsistencySolver=NEWTON_XTOL_AFTER_FTOL  IndexReductionMethod=DerivativeReplacement  DoDC=off  ResidualTolerance=1e-09  ConsistencyTolSource=GLOBAL  ConsistencyAbsTol=0.001  ConsistencyRelTol=0.001  ConsistencyTolFactor=0.001  UseLocalSolver=off  LocalSolverChoice=NE_BACKWARD_EULER_ADVANCER  ResolveIndetEquations=on  FunctionEvalNumThread=1  LocalSolverSampleTime=0.001  DoFixedCost=off  MaxNonlinIter=3  MaxModeIter=2  ComputeImpulses=off  ImpulseIterations=2  LinearAlgebra=auto  LinearAlgebraNumThread=0  EquationFormulation=NE_TIME_EF  DelaysMemoryBudget=1024  AutomaticFiltering=on  FilteringTimeConstant=0.001  PartitionStorageMethod=AS_NEEDED  PartitionMemoryBudget=1024  PartitionMethod=ROBUST  MultibodyUseLocalSolver=off  MultibodyLocalSolverChoice=ODE1  MultibodyLocalSolverSampleTime=0.001
  Terminator : Terminator
  Voltage Sensor1 : fl_lib/Electrical/Electrical Sensors/Voltage Sensor
  Voltage Sensor6 : fl_lib/Electrical/Electrical Sensors/Voltage Sensor
  derivative : TransferFcn  Denominator=[1/wd 1]
  Connection Port1 : PMIOPort  Side=Left
  Connection Port2 : PMIOPort  Port=2  Side=Right
  wires:
  PS-Simulink Converter/1 -> Product/2, Terminator/1  "V_WEC_1"
  PS-Simulink Converter1/1 -> Divide/2, B_rad/1, derivative/1, Integrator/1  "V_1"
  Integrator/1 -> K_hs/1  "eta1"
  K_hs/1 -> Gain/1  "Fhs1"
  B_rad/1 -> Add/2  "Fr1"
  derivative/1 -> M_add/1
  M_add/1 -> Add/3  "Fm_add1"
  Add/1 -> Product/1, Simulink-PS Converter/1  "F_ex1"
  Gain/1 -> Add/1
  Product/1 -> Divide/1  "P_WEC1"
  connections:
  Voltage Sensor6/LConn1 -- Resistor3/LConn1 -- Resistor2/LConn1 -- Resistor1/LConn1 -- Inductor1/LConn1 -- Controlled Current Source/LConn1 -- Capacitor1/LConn1
  PS-Simulink Converter/LConn1 -- Voltage Sensor6/RConn1
  Connection Port1/RConn1 -- Resistor/LConn1 -- Voltage Sensor1/LConn1
  Connection Port2/RConn1 -- Resistor/RConn1 -- Voltage Sensor1/RConn2 -- Electrical Reference2/LConn1
  PS-Simulink Converter1/LConn1 -- Voltage Sensor1/RConn1
  Simulink-PS Converter/RConn1 -- Controlled Current Source/RConn1
  Capacitor1/RConn1 -- Controlled Current Source/RConn2 -- Solver Configuration/RConn1 -- Voltage Sensor6/RConn2 -- Resistor3/RConn1 -- Resistor2/RConn1 -- Resistor1/RConn1 -- Electrical Reference/LConn1 -- Inductor1/RConn1

== system Pi_LUPA/WEC2 ==
  Add : Sum  Inputs=+++
  B_rad : Gain  Gain=1/ckt.R_rad
  Capacitor1 : fl_lib/Electrical/Electrical Elements/Capacitor  c=ckt.C_M F  r=0 Ohm  g=0 1/Ohm  i_specify=off  i_priority=None  i=0 A  i_nominal_specify=off  i_nominal_value=1  i_nominal_unit=A  v_specify=off  v_priority=None  v=0 V  v_nominal_specify=off  v_nominal_value=1  v_nominal_unit=V  vc_specify=off  vc_priority=High  vc=0 V  vc_nominal_specify=off  vc_nominal_value=1  vc_nominal_unit=V
  Controlled Current Source : fl_lib/Electrical/Electrical Sources/Controlled Current Source
  Electrical Reference : fl_lib/Electrical/Electrical Elements/Electrical Reference
  Electrical Reference2 : fl_lib/Electrical/Electrical Elements/Electrical Reference
  Fex_FIR_IRF : Subsystem  Commented=on
  Gain : Gain  Gain=0.65
  Inductor1 : fl_lib/Electrical/Electrical Elements/Inductor  l=ckt.L_hs H  r=0 Ohm  g=0 1/Ohm  i_specify=off  i_priority=None  i=0 A  i_nominal_specify=off  i_nominal_value=1  i_nominal_unit=A  v_specify=off  v_priority=None  v=0 V  v_nominal_specify=off  v_nominal_value=1  v_nominal_unit=V  i_L_specify=off  i_L_priority=High  i_L=0 A  i_L_nominal_specify=off  i_L_nominal_value=1  i_L_nominal_unit=A
  Integrator : Integrator  InitialCondition=-A
  K_hs : Gain  Gain=1/ckt.L_hs
  M_add : Gain  Gain=ckt.C_add
  PS-Simulink Converter : nesl_utility/PS-Simulink Converter  PhysicalDomain=network_engine_domain  SubClassName=ps_output  LeftPortType=input  RightPortType=output  PseudoPeriodic=off  Frequencies=[]  VectorFormat=inherit  Unit=inherit  AffineConversion=off
  PS-Simulink Converter1 : nesl_utility/PS-Simulink Converter  PhysicalDomain=network_engine_domain  SubClassName=ps_output  LeftPortType=input  RightPortType=output  PseudoPeriodic=off  Frequencies=[]  VectorFormat=inherit  Unit=V  AffineConversion=off
  Resistor : fl_lib/Electrical/Electrical Elements/Resistor  R=1.1*1e-3 Ohm  i_specify=off  i_priority=None  i=0 A  i_nominal_specify=off  i_nominal_value=1  i_nominal_unit=A  v_specify=off  v_priority=None  v=0 V  v_nominal_specify=off  v_nominal_value=1  v_nominal_unit=V
  Resistor1 : fl_lib/Electrical/Electrical Elements/Resistor  R=ckt.R_rad Ohm  i_specify=off  i_priority=None  i=0 A  i_nominal_specify=off  i_nominal_value=1  i_nominal_unit=A  v_specify=off  v_priority=None  v=0 V  v_nominal_specify=off  v_nominal_value=1  v_nominal_unit=V
  Resistor2 : fl_lib/Electrical/Electrical Elements/Resistor  R=ckt.R_fric Ohm  i_specify=off  i_priority=None  i=0 A  i_nominal_specify=off  i_nominal_value=1  i_nominal_unit=A  v_specify=off  v_priority=None  v=0 V  v_nominal_specify=off  v_nominal_value=1  v_nominal_unit=V
  Resistor3 : fl_lib/Electrical/Electrical Elements/Resistor  R=ckt.R_pto Ohm  i_specify=off  i_priority=None  i=0 A  i_nominal_specify=off  i_nominal_value=1  i_nominal_unit=A  v_specify=off  v_priority=None  v=0 V  v_nominal_specify=off  v_nominal_value=1  v_nominal_unit=V
  Simulink-PS Converter : nesl_utility/Simulink-PS Converter  PhysicalDomain=network_engine_domain  SubClassName=ps_input  LeftPortType=input  RightPortType=output  PseudoPeriodic=off  Frequencies=[]  NoiseDistribution=none  NoiseParameters=[]  Unit=A  AffineConversion=off  FilteringAndDerivatives=filter  SimscapeFilterOrder=1  InputFilterTimeConstant=0.001  UdotUserProvided=0
  Solver Configuration : nesl_utility/Solver Configuration  PhysicalDomain=network_engine_domain  SubClassName=solver  LeftPortType=input  RightPortType=generic  Tones=[]  Harmonics=[]  SimulateNoise=off  Profile=off  UseLocalSampling=off  EnableSwitchedLinearOptims=on  FrequencyDomain=off  UseCCode=off  RelTol=0.001  AbsTol=0.001  MinStep=1e-09  ToWorkspace=off  RevertToSquareIcSolve=off  NumHomotopyIterations=100  PhasorMode=off  PhasorModeNumHarmonics=1  ConsistencySolver=NEWTON_XTOL_AFTER_FTOL  IndexReductionMethod=DerivativeReplacement  DoDC=off  ResidualTolerance=1e-09  ConsistencyTolSource=GLOBAL  ConsistencyAbsTol=0.001  ConsistencyRelTol=0.001  ConsistencyTolFactor=0.001  UseLocalSolver=off  LocalSolverChoice=NE_BACKWARD_EULER_ADVANCER  ResolveIndetEquations=on  FunctionEvalNumThread=1  LocalSolverSampleTime=0.001  DoFixedCost=off  MaxNonlinIter=3  MaxModeIter=2  ComputeImpulses=off  ImpulseIterations=2  LinearAlgebra=auto  LinearAlgebraNumThread=0  EquationFormulation=NE_TIME_EF  DelaysMemoryBudget=1024  AutomaticFiltering=on  FilteringTimeConstant=0.001  PartitionStorageMethod=AS_NEEDED  PartitionMemoryBudget=1024  PartitionMethod=ROBUST  MultibodyUseLocalSolver=off  MultibodyLocalSolverChoice=ODE1  MultibodyLocalSolverSampleTime=0.001
  Terminator : Terminator
  Voltage Sensor1 : fl_lib/Electrical/Electrical Sensors/Voltage Sensor
  Voltage Sensor6 : fl_lib/Electrical/Electrical Sensors/Voltage Sensor
  derivative : TransferFcn  Denominator=[1/wd 1]
  Connection Port1 : PMIOPort  Side=Left
  Connection Port2 : PMIOPort  Port=2  Side=Right
  wires:
  PS-Simulink Converter/1 -> Terminator/1  "V_WEC_2"
  PS-Simulink Converter1/1 -> Integrator/1, B_rad/1, derivative/1  "V_2"
  Integrator/1 -> K_hs/1  "eta2"
  K_hs/1 -> Gain/1  "Fhs2"
  B_rad/1 -> Add/2  "Fr2"
  derivative/1 -> M_add/1
  M_add/1 -> Add/3  "Fm_add2"
  Add/1 -> Simulink-PS Converter/1  "F_ex2"
  Gain/1 -> Add/1
  connections:
  Voltage Sensor6/LConn1 -- Resistor3/LConn1 -- Resistor2/LConn1 -- Resistor1/LConn1 -- Inductor1/LConn1 -- Controlled Current Source/LConn1 -- Capacitor1/LConn1
  PS-Simulink Converter/LConn1 -- Voltage Sensor6/RConn1
  Connection Port1/RConn1 -- Resistor/LConn1 -- Voltage Sensor1/LConn1
  Voltage Sensor1/RConn2 -- Resistor/RConn1 -- Connection Port2/RConn1 -- Electrical Reference2/LConn1
  PS-Simulink Converter1/LConn1 -- Voltage Sensor1/RConn1
  Simulink-PS Converter/RConn1 -- Controlled Current Source/RConn1
  Capacitor1/RConn1 -- Voltage Sensor6/RConn2 -- Resistor3/RConn1 -- Resistor2/RConn1 -- Resistor1/RConn1 -- Electrical Reference/LConn1 -- Inductor1/RConn1 -- Controlled Current Source/RConn2 -- Solver Configuration/RConn1
